simulink model "solar"  (R2021a)
settings: Solver=ode45  StartTime=0.0  StopTime=10  MaxStep=1  RelTol=1e-3  AbsTol=1e-6
libraries: spsSeriesRLCBranchLib x3, spsDiodeLib x1, spsIGBTLib x1, spsPVArrayLib x1, spsVoltageMeasurementLib x1
settings Model: Creator=Udana  LastModifiedBy=Udana
settings SolverCC: AlgebraicLoopSolver=TrustRegion

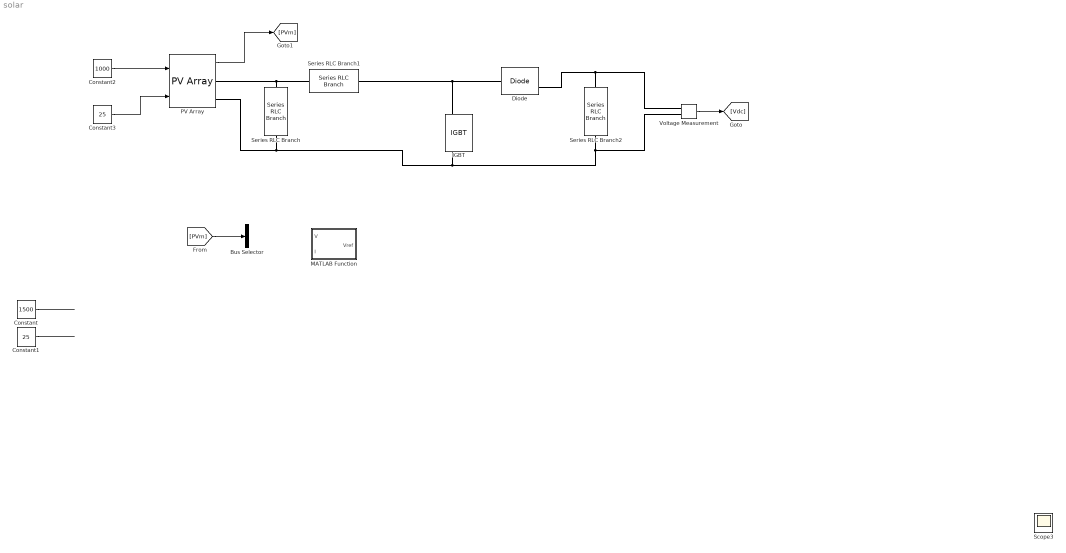
== system solar ==
  Bus Selector : BusSelector  OutputSignals=V_PV,I_PV
  Constant : Constant  Value=1500
  Constant1 : Constant  Value=25
  Constant2 : Constant  Value=1000
  Constant3 : Constant  Value=25
  Diode : spsDiodeLib/Diode  Ron=0.001  Lon=0  Vf=0.8  IC=0  UseSnubber=0  Rs=500  Cs=250e-9  Measurements=on
  IGBT : spsIGBTLib/IGBT  Ron=0.001  Lon=0  Vf=1  Tf=1e-6  Tt=2e-6  IC=0  Rs=1e5  Cs=inf  Measurements=on
  MATLAB Function : MATLAB Function  TreatAsAtomicUnit=on
  PV Array : spsPVArrayLib/PV Array  Npar=11  Nser=11  PlotType=array @ 25 deg.C & specified irradiances  S_vec="[ 1000  500  100 ]"  Temp_C_vec="[ 45 25  ]"  ModuleName=Advance Solar Hydro Wind Power API156P-210  PlotWhenSelected=off  Pm=209.948  Ncell=60  Voc=36.4  Isc=7.86  Vm=29.2  Im=7.19  beta_Voc_pc=-0.3651  alpha_Isc_pc=0.075  beta_Voc=-0.1329  alpha_Isc=0.005895  IL=7.8878  I0=3.2141e-10  nI=0.98883  Rsh=107.0785  Rs=0.37844  RobustModel=off  RobustCellTemperature=313.3991  BAL=on  Tc=1e-6  Tfilter=5e-5
  Scope3 : Scope
  Series RLC Branch : spsSeriesRLCBranchLib/Series RLC Branch  LConnTagsString=__new0  RConnTagsString=__new0  BranchType=C  Resistance=1  Inductance=1e-3  SetiL0=off  InitialCurrent=0  Capacitance=1e-6  Setx0=off  InitialVoltage=0  Measurements=None
  Series RLC Branch1 : spsSeriesRLCBranchLib/Series RLC Branch  LConnTagsString=__new0  RConnTagsString=__new0  BranchType=L  Resistance=1  Inductance=1e-3  SetiL0=off  InitialCurrent=0  Capacitance=1e-6  Setx0=off  InitialVoltage=0  Measurements=None
  Series RLC Branch2 : spsSeriesRLCBranchLib/Series RLC Branch  LConnTagsString=__new0  RConnTagsString=__new0  BranchType=C  Resistance=1  Inductance=1e-3  SetiL0=off  InitialCurrent=0  Capacitance=1e-6  Setx0=off  InitialVoltage=0  Measurements=None
  Voltage Measurement : spsVoltageMeasurementLib/Voltage Measurement  PhasorSimulation=off  OutputType=Complex  PSBequivalent=0
  wires:
  Constant1/1 -> ?
  Constant/1 -> ?
  Constant2/1 -> PV Array/1
  Constant3/1 -> PV Array/2
  Voltage Measurement/1 -> [Vdc]
  PV Array/1 -> [PVm]
  [PVm] -> Bus Selector/1
  connections:
  PV Array/RConn1 -- Series RLC Branch1/RConn1 -- Series RLC Branch/LConn1
  Series RLC Branch/RConn1 -- Voltage Measurement/LConn2 -- Series RLC Branch2/RConn1 -- IGBT/RConn1 -- PV Array/RConn2
  Series RLC Branch1/LConn1 -- Diode/LConn1 -- IGBT/LConn1
  Diode/RConn1 -- Voltage Measurement/LConn1 -- Series RLC Branch2/LConn1

== matlab function solar/MATLAB Function ==
  data: V input; Vref output; I input
function Vref = mppt(V, I)

Vinit=0.42
Vmax=0.9
Vmin=0.1
